simulink model "smith"  (Simulink 8.3)
settings: Solver=ode45  StartTime=0.0  StopTime=150  MaxStep=0.01  RelTol=1e-3
settings Model: Creator=thinkpad  LastModifiedBy=York
settings OptimizationCC: ExpressionDepthLimit=2147483647  InitFltsAndDblsToZero=on
settings DebuggingCC: SaveWithParameterizedLinksMsg=none  SignalResolutionControl=TryResolveAllWithWarning  MultiTaskDSMMsg=warning  MultiTaskCondExecSysMsg=none  FcnCallInpInsideContextMsg=UseLocalSettings
settings RTWCC: IncludeERTFirstTime=on
settings GRTTargetCC: TargetFcnLib=ansi_tfl_tmw.mat

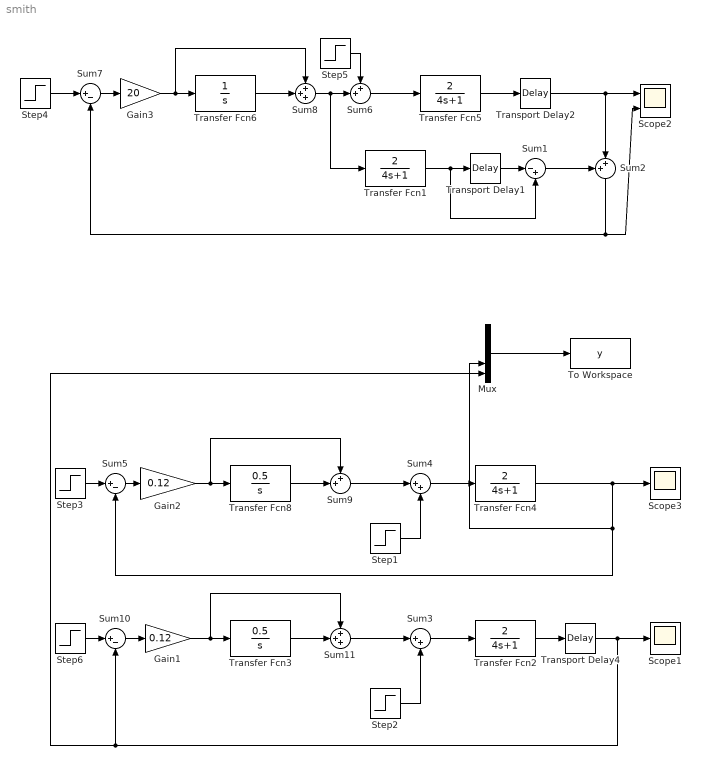
== system smith ==
  Gain1 : Gain  Gain=0.12
  Gain2 : Gain  Gain=0.12
  Gain3 : Gain  Gain=20
  Mux : Mux  Inputs=5
  Scope1 : Scope
      settings: TimeRange=150  SaveName=ScopeData2
  Scope2 : Scope  NumInputPorts=2
      settings: TimeRange=50  YMin=0~-5  YMax=14~5
  Scope3 : Scope
  Step1 : Step  Time=65  SampleTime=0
  Step2 : Step  Time=65  SampleTime=0
  Step3 : Step  Time=0  SampleTime=0
  Step4 : Step  Time=0  SampleTime=0
  Step5 : Step  Time=10  SampleTime=0
  Step6 : Step  Time=0  SampleTime=0
  Sum1 : Sum  Inputs=|-+
  Sum10 : Sum  Inputs=|+-
  Sum11 : Sum  Inputs=+++
  Sum2 : Sum  Inputs=++|
  Sum3 : Sum  Inputs=|++
  Sum4 : Sum  Inputs=|++
  Sum5 : Sum  Inputs=|+-
  Sum6 : Sum  Inputs=++|
  Sum7 : Sum  Inputs=|+-
  Sum8 : Sum  Inputs=+++
  Sum9 : Sum  Inputs=++|
  To Workspace : ToWorkspace  VariableName=y  SaveFormat=Structure With Time  SampleTime=-1
  Transfer Fcn{1..2,4..5} (4 alike) : TransferFcn  Numerator=[2]  Denominator=[4 1]
  Transfer Fcn3 : TransferFcn  Numerator=[0.5]  Denominator=[1 0]
  Transfer Fcn6 : TransferFcn  Denominator=[1 0]
  Transfer Fcn8 : TransferFcn  Numerator=[0.5]  Denominator=[1 0]
  Transport Delay1 : TransportDelay  DelayTime=4
  Transport Delay2 : TransportDelay  DelayTime=4  BufferSize=10240
  Transport Delay4 : TransportDelay  DelayTime=4  BufferSize=10240
  wires:
  Transfer Fcn5/1 -> Transport Delay2/1
  Transport Delay2/1 -> Sum2/2, Scope2/1
  Sum6/1 -> Transfer Fcn5/1
  Step4/1 -> Sum7/1
  Gain3/1 -> Transfer Fcn6/1, Sum8/1
  Sum7/1 -> Gain3/1
  Sum8/1 -> Sum6/2, Transfer Fcn1/1
  Step5/1 -> Sum6/1
  Transfer Fcn6/1 -> Sum8/2
  Transport Delay1/1 -> Sum1/1
  Transfer Fcn1/1 -> Transport Delay1/1, Sum1/2
  Sum1/1 -> Sum2/1
  Sum2/1 -> Sum7/2, Scope2/2
  Sum4/1 -> Transfer Fcn4/1
  Step3/1 -> Sum5/1
  Gain2/1 -> Transfer Fcn8/1, Sum9/1
  Sum5/1 -> Gain2/1
  Sum9/1 -> Sum4/1
  Transfer Fcn8/1 -> Sum9/2
  Mux/1 -> To Workspace/1
  Step1/1 -> Sum4/2
  Transfer Fcn4/1 -> Mux/4, Sum5/2, Scope3/1
  Transfer Fcn2/1 -> Transport Delay4/1
  Sum3/1 -> Transfer Fcn2/1
  Step6/1 -> Sum10/1
  Gain1/1 -> Transfer Fcn3/1, Sum11/1
  Transfer Fcn3/1 -> Sum11/2
  Step2/1 -> Sum3/2
  Transport Delay4/1 -> Scope1/1, Mux/5, Sum10/2
  Sum11/1 -> Sum3/1
  Sum10/1 -> Gain1/1
